simulink model "TestStructure"  (R2023b)
settings: Solver=FixedStepDiscrete  StartTime=0.0  StopTime=inf  FixedStep=SampleTime  RelTol=1e-3
InitFcn:
  | SampleTime = 0.001;
  | ButtonValue=0;
  | load("BusConfig.mat");
undefined symbols (not defined in the file): DiscIntNeverNeededParam
libraries: slrealtimeethercatlib x219, dspfdesign x28, dspstat3 x23, simulink x21, slpidlib x10, dspswit3 x8, commfilt2 x2, dspsigops x1
(part 6 of 8)

== system TestStructure/Bus/Subsystem6/Subsystem/Subsystem11 ==
  EtherCAT PDO Receive1 : slrealtimeethercatlib/EtherCAT PDO Receive  Priority=2  sig_name=Box 1 (PIC32 EtherCAT Slave01).INPUTS process data mapping.FORCE1  sig_offset=696  sig_type=single  type_size=32  sig_dim=1  device_id=0  sample_time=0.001000
  EtherCAT PDO Receive2 : slrealtimeethercatlib/EtherCAT PDO Receive  Priority=2  sig_name=Box 1 (PIC32 EtherCAT Slave01).INPUTS process data mapping.FORCE2  sig_offset=728  sig_type=single  type_size=32  sig_dim=1  device_id=0  sample_time=0.001000
  EtherCAT PDO Receive3 : slrealtimeethercatlib/EtherCAT PDO Receive  Priority=2  sig_name=Box 1 (PIC32 EtherCAT Slave01).INPUTS process data mapping.IMU1_X  sig_offset=952  sig_type=single  type_size=32  sig_dim=1  device_id=0  sample_time=0.001000
  EtherCAT PDO Receive4 : slrealtimeethercatlib/EtherCAT PDO Receive  Priority=2  sig_name=Box 1 (PIC32 EtherCAT Slave01).INPUTS process data mapping.IMU1_Y  sig_offset=984  sig_type=single  type_size=32  sig_dim=1  device_id=0  sample_time=0.001000
  EtherCAT PDO Receive5 : slrealtimeethercatlib/EtherCAT PDO Receive  Priority=2  sig_name=Box 1 (PIC32 EtherCAT Slave01).INPUTS process data mapping.IMU1_Z  sig_offset=1016  sig_type=single  type_size=32  sig_dim=1  device_id=0  sample_time=0.001000
  EtherCAT PDO Receive6 : slrealtimeethercatlib/EtherCAT PDO Receive  Priority=2  sig_name=Box 1 (PIC32 EtherCAT Slave01).INPUTS process data mapping.IMU2_X  sig_offset=1048  sig_type=single  type_size=32  sig_dim=1  device_id=0  sample_time=0.001000
  EtherCAT PDO Receive7 : slrealtimeethercatlib/EtherCAT PDO Receive  Priority=2  sig_name=Box 1 (PIC32 EtherCAT Slave01).INPUTS process data mapping.FORCE3  sig_offset=760  sig_type=single  type_size=32  sig_dim=1  device_id=0  sample_time=0.001000
  Out1 : Outport
  Out2 : Outport  Port=2
  Out3 : Outport  Port=3
  Out4 : Outport  Port=4
  Out5 : Outport  Port=5
  Out6 : Outport  Port=6
  Out7 : Outport  Port=7
  wires:
  EtherCAT PDO Receive1/1 -> Out1/1
  EtherCAT PDO Receive2/1 -> Out2/1
  EtherCAT PDO Receive3/1 -> Out3/1
  EtherCAT PDO Receive4/1 -> Out4/1
  EtherCAT PDO Receive5/1 -> Out5/1
  EtherCAT PDO Receive6/1 -> Out6/1
  EtherCAT PDO Receive7/1 -> Out7/1

== system TestStructure/Bus/Subsystem6/Subsystem/Subsystem2 ==
  In1 : Inport
  EtherCAT PDO Receive1 : slrealtimeethercatlib/EtherCAT PDO Receive  Priority=2  sig_name=Drive 6 (Elmo Drive ).Inputs.Position actual value  sig_offset=13232  sig_type=int32  type_size=32  sig_dim=1  device_id=0  sample_time=0.001000
  EtherCAT PDO Receive2 : slrealtimeethercatlib/EtherCAT PDO Receive  Priority=2  sig_name=Drive 6 (Elmo Drive ).Inputs_1.Velocity actual value  sig_offset=13312  sig_type=int32  type_size=32  sig_dim=1  device_id=0  sample_time=0.001000
  EtherCAT PDO Receive3 : slrealtimeethercatlib/EtherCAT PDO Receive  Priority=2  sig_name=Drive 6 (Elmo Drive ).Inputs.Torque actual value  sig_offset=13264  sig_type=int16  type_size=16  sig_dim=1  device_id=0  sample_time=0.001000
  EtherCAT PDO Receive4 : slrealtimeethercatlib/EtherCAT PDO Receive  Priority=2  sig_name=Drive 6 (Elmo Drive ).Inputs_2.DC link circuit voltage  sig_offset=13344  sig_type=uint32  type_size=32  sig_dim=1  device_id=0  sample_time=0.001000
  EtherCAT PDO Receive5 : slrealtimeethercatlib/EtherCAT PDO Receive  Priority=2  sig_name=Drive 6 (Elmo Drive ).Inputs.Mode of operation display  sig_offset=13296  sig_type=int8  type_size=8  sig_dim=1  device_id=0  sample_time=0.001000
  EtherCAT PDO Transmit : slrealtimeethercatlib/EtherCAT PDO Transmit  Priority=5  Commented=on  sig_name=Drive 4 (Elmo Drive ).Outputs.Target Torque  sig_offset=37072  sig_type=int16  type_size=16  sig_dim=1  device_id=0  sample_time=0.001000
  Out1 : Outport
  Out2 : Outport  Port=2
  Out3 : Outport  Port=3
  Out4 : Outport  Port=4
  Out5 : Outport  Port=5
  wires:
  In1/1 -> EtherCAT PDO Transmit/1
  EtherCAT PDO Receive5/1 -> Out5/1
  EtherCAT PDO Receive4/1 -> Out4/1
  EtherCAT PDO Receive3/1 -> Out3/1
  EtherCAT PDO Receive2/1 -> Out2/1
  EtherCAT PDO Receive1/1 -> Out1/1

== system TestStructure/Bus/Subsystem6/Subsystem/Subsystem3 ==
  In1 : Inport
  EtherCAT PDO Receive1 : slrealtimeethercatlib/EtherCAT PDO Receive  Priority=2  sig_name=Drive 2 (Elmo Drive ).Inputs.Position actual value  sig_offset=12496  sig_type=int32  type_size=32  sig_dim=1  device_id=0  sample_time=0.001000
  EtherCAT PDO Receive2 : slrealtimeethercatlib/EtherCAT PDO Receive  Priority=2  sig_name=Drive 2 (Elmo Drive ).Inputs_1.Velocity actual value  sig_offset=12576  sig_type=int32  type_size=32  sig_dim=1  device_id=0  sample_time=0.001000
  EtherCAT PDO Receive3 : slrealtimeethercatlib/EtherCAT PDO Receive  Priority=2  sig_name=Drive 2 (Elmo Drive ).Inputs.Torque actual value  sig_offset=12528  sig_type=int16  type_size=16  sig_dim=1  device_id=0  sample_time=0.001000
  EtherCAT PDO Receive4 : slrealtimeethercatlib/EtherCAT PDO Receive  Priority=2  sig_name=Drive 2 (Elmo Drive ).Inputs_2.DC link circuit voltage  sig_offset=12608  sig_type=uint32  type_size=32  sig_dim=1  device_id=0  sample_time=0.001000
  EtherCAT PDO Receive5 : slrealtimeethercatlib/EtherCAT PDO Receive  Priority=2  sig_name=Drive 2 (Elmo Drive ).Inputs.Mode of operation display  sig_offset=12560  sig_type=int8  type_size=8  sig_dim=1  device_id=0  sample_time=0.001000
  EtherCAT PDO Transmit : slrealtimeethercatlib/EtherCAT PDO Transmit  Priority=5  sig_name=Drive 2 (Elmo Drive ).Outputs.Target Torque  sig_offset=12496  sig_type=int16  type_size=16  sig_dim=1  device_id=0  sample_time=0.001000
  Out1 : Outport
  Out2 : Outport  Port=2
  Out3 : Outport  Port=3
  Out4 : Outport  Port=4
  Out5 : Outport  Port=5
  wires:
  In1/1 -> EtherCAT PDO Transmit/1
  EtherCAT PDO Receive5/1 -> Out5/1
  EtherCAT PDO Receive4/1 -> Out4/1
  EtherCAT PDO Receive3/1 -> Out3/1
  EtherCAT PDO Receive2/1 -> Out2/1
  EtherCAT PDO Receive1/1 -> Out1/1

== system TestStructure/Bus/Subsystem6/Subsystem/Subsystem4 ==
  In1 : Inport
  EtherCAT PDO Receive1 : slrealtimeethercatlib/EtherCAT PDO Receive  Priority=2  sig_name=Drive 2 (Elmo Drive ).Inputs.Position actual value  sig_offset=12496  sig_type=int32  type_size=32  sig_dim=1  device_id=0  sample_time=0.001000
  EtherCAT PDO Receive2 : slrealtimeethercatlib/EtherCAT PDO Receive  Priority=2  sig_name=Drive 2 (Elmo Drive ).Inputs_1.Velocity actual value  sig_offset=12576  sig_type=int32  type_size=32  sig_dim=1  device_id=0  sample_time=0.001000
  EtherCAT PDO Receive3 : slrealtimeethercatlib/EtherCAT PDO Receive  Priority=2  sig_name=Drive 2 (Elmo Drive ).Inputs.Torque actual value  sig_offset=12528  sig_type=int16  type_size=16  sig_dim=1  device_id=0  sample_time=0.001000
  EtherCAT PDO Receive4 : slrealtimeethercatlib/EtherCAT PDO Receive  Priority=2  sig_name=Drive 2 (Elmo Drive ).Inputs_2.DC link circuit voltage  sig_offset=12608  sig_type=uint32  type_size=32  sig_dim=1  device_id=0  sample_time=0.001000
  EtherCAT PDO Receive5 : slrealtimeethercatlib/EtherCAT PDO Receive  Priority=2  sig_name=Drive 2 (Elmo Drive ).Inputs.Mode of operation display  sig_offset=12560  sig_type=int8  type_size=8  sig_dim=1  device_id=0  sample_time=0.001000
  EtherCAT PDO Transmit : slrealtimeethercatlib/EtherCAT PDO Transmit  Priority=5  sig_name=Drive 2 (Elmo Drive ).Outputs.Target Torque  sig_offset=12496  sig_type=int16  type_size=16  sig_dim=1  device_id=0  sample_time=0.001000
  Out1 : Outport
  Out2 : Outport  Port=2
  Out3 : Outport  Port=3
  Out4 : Outport  Port=4
  Out5 : Outport  Port=5
  wires:
  In1/1 -> EtherCAT PDO Transmit/1
  EtherCAT PDO Receive5/1 -> Out5/1
  EtherCAT PDO Receive4/1 -> Out4/1
  EtherCAT PDO Receive3/1 -> Out3/1
  EtherCAT PDO Receive2/1 -> Out2/1
  EtherCAT PDO Receive1/1 -> Out1/1

== system TestStructure/Bus/Subsystem6/Subsystem/Subsystem5 ==
  EtherCAT PDO Receive1 : slrealtimeethercatlib/EtherCAT PDO Receive  Priority=2  sig_name=Box 2 (PIC32 EtherCAT Slave01).INPUTS process data mapping.FORCE1  sig_offset=696  sig_type=single  type_size=32  sig_dim=1  device_id=0  sample_time=0.001000
  EtherCAT PDO Receive{2..6} (5 alike) : slrealtimeethercatlib/EtherCAT PDO Receive  Priority=2  Commented=on  sig_name=Uninitialized Block  sig_offset=1  sig_type=boolean  type_size=1  sig_dim=1  device_id=0  sample_time=1
  EtherCAT PDO Receive7 : slrealtimeethercatlib/EtherCAT PDO Receive  Priority=2  sig_name=Box 2 (PIC32 EtherCAT Slave01).INPUTS process data mapping.FORCE3  sig_offset=760  sig_type=single  type_size=32  sig_dim=1  device_id=0  sample_time=0.001000
  Out1 : Outport
  Out2 : Outport  Port=2
  Out3 : Outport  Port=3
  Out4 : Outport  Port=4
  Out5 : Outport  Port=5
  Out6 : Outport  Port=6
  Out7 : Outport  Port=7
  wires:
  EtherCAT PDO Receive1/1 -> Out1/1
  EtherCAT PDO Receive2/1 -> Out2/1
  EtherCAT PDO Receive3/1 -> Out3/1
  EtherCAT PDO Receive4/1 -> Out4/1
  EtherCAT PDO Receive5/1 -> Out5/1
  EtherCAT PDO Receive6/1 -> Out6/1
  EtherCAT PDO Receive7/1 -> Out7/1

== system TestStructure/Bus/Subsystem6/Subsystem/Subsystem6 ==
  EtherCAT PDO Receive1 : slrealtimeethercatlib/EtherCAT PDO Receive  Priority=2  sig_name=Box 5 (PIC32 EtherCAT Slave01).INPUTS process data mapping.FORCE1  sig_offset=12496  sig_type=single  type_size=32  sig_dim=1  device_id=0  sample_time=0.001000
  EtherCAT PDO Receive2 : slrealtimeethercatlib/EtherCAT PDO Receive  Priority=2  Commented=on  sig_name=Box 6 (PIC32 EtherCAT Slave01).INPUTS process data mapping.FORCE2  sig_offset=37104  sig_type=single  type_size=32  sig_dim=1  device_id=0  sample_time=0.001000
  EtherCAT PDO Receive3 : slrealtimeethercatlib/EtherCAT PDO Receive  Priority=2  Commented=on  sig_name=Box 6 (PIC32 EtherCAT Slave01).INPUTS process data mapping.IMU1_X  sig_offset=37328  sig_type=single  type_size=32  sig_dim=1  device_id=0  sample_time=0.001000
  EtherCAT PDO Receive4 : slrealtimeethercatlib/EtherCAT PDO Receive  Priority=2  Commented=on  sig_name=Box 6 (PIC32 EtherCAT Slave01).INPUTS process data mapping.IMU1_Y  sig_offset=37360  sig_type=single  type_size=32  sig_dim=1  device_id=0  sample_time=0.001000
  EtherCAT PDO Receive5 : slrealtimeethercatlib/EtherCAT PDO Receive  Priority=2  Commented=on  sig_name=Box 6 (PIC32 EtherCAT Slave01).INPUTS process data mapping.IMU1_Z  sig_offset=37392  sig_type=single  type_size=32  sig_dim=1  device_id=0  sample_time=0.001000
  EtherCAT PDO Receive6 : slrealtimeethercatlib/EtherCAT PDO Receive  Priority=2  Commented=on  sig_name=Box 6 (PIC32 EtherCAT Slave01).INPUTS process data mapping.IMU2_X  sig_offset=37424  sig_type=single  type_size=32  sig_dim=1  device_id=0  sample_time=0.001000
  EtherCAT PDO Receive7 : slrealtimeethercatlib/EtherCAT PDO Receive  Priority=2  sig_name=Box 5 (PIC32 EtherCAT Slave01).INPUTS process data mapping.FORCE3  sig_offset=12560  sig_type=single  type_size=32  sig_dim=1  device_id=0  sample_time=0.001000
  Out1 : Outport
  Out2 : Outport  Port=2
  Out3 : Outport  Port=3
  Out4 : Outport  Port=4
  Out5 : Outport  Port=5
  Out6 : Outport  Port=6
  Out7 : Outport  Port=7
  wires:
  EtherCAT PDO Receive1/1 -> Out1/1
  EtherCAT PDO Receive2/1 -> Out2/1
  EtherCAT PDO Receive3/1 -> Out3/1
  EtherCAT PDO Receive4/1 -> Out4/1
  EtherCAT PDO Receive5/1 -> Out5/1
  EtherCAT PDO Receive6/1 -> Out6/1
  EtherCAT PDO Receive7/1 -> Out7/1

== system TestStructure/Bus/Subsystem6/Subsystem/Subsystem7 ==
  EtherCAT PDO Receive1 : slrealtimeethercatlib/EtherCAT PDO Receive  Priority=2  sig_name=Box 1 (PIC32 EtherCAT Slave01).INPUTS process data mapping.FORCE1  sig_offset=696  sig_type=single  type_size=32  sig_dim=1  device_id=0  sample_time=0.001000
  EtherCAT PDO Receive2 : slrealtimeethercatlib/EtherCAT PDO Receive  Priority=2  sig_name=Box 1 (PIC32 EtherCAT Slave01).INPUTS process data mapping.FORCE2  sig_offset=728  sig_type=single  type_size=32  sig_dim=1  device_id=0  sample_time=0.001000
  EtherCAT PDO Receive3 : slrealtimeethercatlib/EtherCAT PDO Receive  Priority=2  sig_name=Box 1 (PIC32 EtherCAT Slave01).INPUTS process data mapping.IMU1_X  sig_offset=952  sig_type=single  type_size=32  sig_dim=1  device_id=0  sample_time=0.001000
  EtherCAT PDO Receive4 : slrealtimeethercatlib/EtherCAT PDO Receive  Priority=2  sig_name=Box 1 (PIC32 EtherCAT Slave01).INPUTS process data mapping.IMU1_Y  sig_offset=984  sig_type=single  type_size=32  sig_dim=1  device_id=0  sample_time=0.001000
  EtherCAT PDO Receive5 : slrealtimeethercatlib/EtherCAT PDO Receive  Priority=2  sig_name=Box 1 (PIC32 EtherCAT Slave01).INPUTS process data mapping.IMU1_Z  sig_offset=1016  sig_type=single  type_size=32  sig_dim=1  device_id=0  sample_time=0.001000
  EtherCAT PDO Receive6 : slrealtimeethercatlib/EtherCAT PDO Receive  Priority=2  sig_name=Box 1 (PIC32 EtherCAT Slave01).INPUTS process data mapping.IMU2_X  sig_offset=1048  sig_type=single  type_size=32  sig_dim=1  device_id=0  sample_time=0.001000
  EtherCAT PDO Receive7 : slrealtimeethercatlib/EtherCAT PDO Receive  Priority=2  sig_name=Box 1 (PIC32 EtherCAT Slave01).INPUTS process data mapping.FORCE3  sig_offset=760  sig_type=single  type_size=32  sig_dim=1  device_id=0  sample_time=0.001000
  Out1 : Outport
  Out2 : Outport  Port=2
  Out3 : Outport  Port=3
  Out4 : Outport  Port=4
  Out5 : Outport  Port=5
  Out6 : Outport  Port=6
  Out7 : Outport  Port=7
  wires:
  EtherCAT PDO Receive1/1 -> Out1/1
  EtherCAT PDO Receive2/1 -> Out2/1
  EtherCAT PDO Receive3/1 -> Out3/1
  EtherCAT PDO Receive4/1 -> Out4/1
  EtherCAT PDO Receive5/1 -> Out5/1
  EtherCAT PDO Receive6/1 -> Out6/1
  EtherCAT PDO Receive7/1 -> Out7/1

== system TestStructure/Bus/Subsystem6/Subsystem/Subsystem8 ==
  EtherCAT PDO Receive1 : slrealtimeethercatlib/EtherCAT PDO Receive  Priority=2  sig_name=Box 1 (PIC32 EtherCAT Slave01).INPUTS process data mapping.FORCE1  sig_offset=696  sig_type=single  type_size=32  sig_dim=1  device_id=0  sample_time=0.001000
  EtherCAT PDO Receive2 : slrealtimeethercatlib/EtherCAT PDO Receive  Priority=2  sig_name=Box 1 (PIC32 EtherCAT Slave01).INPUTS process data mapping.FORCE2  sig_offset=728  sig_type=single  type_size=32  sig_dim=1  device_id=0  sample_time=0.001000
  EtherCAT PDO Receive3 : slrealtimeethercatlib/EtherCAT PDO Receive  Priority=2  sig_name=Box 1 (PIC32 EtherCAT Slave01).INPUTS process data mapping.IMU1_X  sig_offset=952  sig_type=single  type_size=32  sig_dim=1  device_id=0  sample_time=0.001000
  EtherCAT PDO Receive4 : slrealtimeethercatlib/EtherCAT PDO Receive  Priority=2  sig_name=Box 1 (PIC32 EtherCAT Slave01).INPUTS process data mapping.IMU1_Y  sig_offset=984  sig_type=single  type_size=32  sig_dim=1  device_id=0  sample_time=0.001000
  EtherCAT PDO Receive5 : slrealtimeethercatlib/EtherCAT PDO Receive  Priority=2  sig_name=Box 1 (PIC32 EtherCAT Slave01).INPUTS process data mapping.IMU1_Z  sig_offset=1016  sig_type=single  type_size=32  sig_dim=1  device_id=0  sample_time=0.001000
  EtherCAT PDO Receive6 : slrealtimeethercatlib/EtherCAT PDO Receive  Priority=2  sig_name=Box 1 (PIC32 EtherCAT Slave01).INPUTS process data mapping.IMU2_X  sig_offset=1048  sig_type=single  type_size=32  sig_dim=1  device_id=0  sample_time=0.001000
  EtherCAT PDO Receive7 : slrealtimeethercatlib/EtherCAT PDO Receive  Priority=2  sig_name=Box 1 (PIC32 EtherCAT Slave01).INPUTS process data mapping.FORCE3  sig_offset=760  sig_type=single  type_size=32  sig_dim=1  device_id=0  sample_time=0.001000
  Out1 : Outport
  Out2 : Outport  Port=2
  Out3 : Outport  Port=3
  Out4 : Outport  Port=4
  Out5 : Outport  Port=5
  Out6 : Outport  Port=6
  Out7 : Outport  Port=7
  wires:
  EtherCAT PDO Receive1/1 -> Out1/1
  EtherCAT PDO Receive2/1 -> Out2/1
  EtherCAT PDO Receive3/1 -> Out3/1
  EtherCAT PDO Receive4/1 -> Out4/1
  EtherCAT PDO Receive5/1 -> Out5/1
  EtherCAT PDO Receive6/1 -> Out6/1
  EtherCAT PDO Receive7/1 -> Out7/1

== system TestStructure/Bus/Subsystem6/Subsystem/Subsystem9 ==
  EtherCAT PDO Receive1 : slrealtimeethercatlib/EtherCAT PDO Receive  Priority=2  sig_name=Box 1 (PIC32 EtherCAT Slave01).INPUTS process data mapping.FORCE1  sig_offset=696  sig_type=single  type_size=32  sig_dim=1  device_id=0  sample_time=0.001000
  EtherCAT PDO Receive2 : slrealtimeethercatlib/EtherCAT PDO Receive  Priority=2  sig_name=Box 1 (PIC32 EtherCAT Slave01).INPUTS process data mapping.FORCE2  sig_offset=728  sig_type=single  type_size=32  sig_dim=1  device_id=0  sample_time=0.001000
  EtherCAT PDO Receive3 : slrealtimeethercatlib/EtherCAT PDO Receive  Priority=2  sig_name=Box 1 (PIC32 EtherCAT Slave01).INPUTS process data mapping.IMU1_X  sig_offset=952  sig_type=single  type_size=32  sig_dim=1  device_id=0  sample_time=0.001000
  EtherCAT PDO Receive4 : slrealtimeethercatlib/EtherCAT PDO Receive  Priority=2  sig_name=Box 1 (PIC32 EtherCAT Slave01).INPUTS process data mapping.IMU1_Y  sig_offset=984  sig_type=single  type_size=32  sig_dim=1  device_id=0  sample_time=0.001000
  EtherCAT PDO Receive5 : slrealtimeethercatlib/EtherCAT PDO Receive  Priority=2  sig_name=Box 1 (PIC32 EtherCAT Slave01).INPUTS process data mapping.IMU1_Z  sig_offset=1016  sig_type=single  type_size=32  sig_dim=1  device_id=0  sample_time=0.001000
  EtherCAT PDO Receive6 : slrealtimeethercatlib/EtherCAT PDO Receive  Priority=2  sig_name=Box 1 (PIC32 EtherCAT Slave01).INPUTS process data mapping.IMU2_X  sig_offset=1048  sig_type=single  type_size=32  sig_dim=1  device_id=0  sample_time=0.001000
  EtherCAT PDO Receive7 : slrealtimeethercatlib/EtherCAT PDO Receive  Priority=2  sig_name=Box 1 (PIC32 EtherCAT Slave01).INPUTS process data mapping.FORCE3  sig_offset=760  sig_type=single  type_size=32  sig_dim=1  device_id=0  sample_time=0.001000
  Out1 : Outport
  Out2 : Outport  Port=2
  Out3 : Outport  Port=3
  Out4 : Outport  Port=4
  Out5 : Outport  Port=5
  Out6 : Outport  Port=6
  Out7 : Outport  Port=7
  wires:
  EtherCAT PDO Receive1/1 -> Out1/1
  EtherCAT PDO Receive2/1 -> Out2/1
  EtherCAT PDO Receive3/1 -> Out3/1
  EtherCAT PDO Receive4/1 -> Out4/1
  EtherCAT PDO Receive5/1 -> Out5/1
  EtherCAT PDO Receive6/1 -> Out6/1
  EtherCAT PDO Receive7/1 -> Out7/1

== system TestStructure/Bus/Subsystem6/Subsystem2/Subsystem7 ==
  EtherCAT PDO Receive1 : slrealtimeethercatlib/EtherCAT PDO Receive  Priority=2  sig_name=Box 8 (PIC32 EtherCAT Slave01).INPUTS process data mapping.FORCE1  sig_offset=24784  sig_type=single  type_size=32  sig_dim=1  device_id=0  sample_time=0.001000
  EtherCAT PDO Receive2 : slrealtimeethercatlib/EtherCAT PDO Receive  Priority=2  sig_name=Box 8 (PIC32 EtherCAT Slave01).INPUTS process data mapping.FORCE2  sig_offset=24816  sig_type=single  type_size=32  sig_dim=1  device_id=0  sample_time=0.001000
  EtherCAT PDO Receive3 : slrealtimeethercatlib/EtherCAT PDO Receive  Priority=2  sig_name=Box 8 (PIC32 EtherCAT Slave01).INPUTS process data mapping.FORCE3  sig_offset=24848  sig_type=single  type_size=32  sig_dim=1  device_id=0  sample_time=0.001000
  EtherCAT PDO Receive4 : slrealtimeethercatlib/EtherCAT PDO Receive  Priority=2  sig_name=Box 8 (PIC32 EtherCAT Slave01).INPUTS process data mapping.FORCE4  sig_offset=24880  sig_type=single  type_size=32  sig_dim=1  device_id=0  sample_time=0.001000
  EtherCAT PDO Receive7 : slrealtimeethercatlib/EtherCAT PDO Receive  Priority=2  Commented=on  sig_name=Box 2 (PIC32 EtherCAT Slave01).INPUTS process data mapping.FORCE5  sig_offset=824  sig_type=single  type_size=32  sig_dim=1  device_id=0  sample_time=0.001000
  Out1 : Outport
  Out2 : Outport  Port=2
  Out3 : Outport  Port=3
  Out4 : Outport  Port=4
  Out7 : Outport  Port=5
  wires:
  EtherCAT PDO Receive1/1 -> Out1/1
  EtherCAT PDO Receive2/1 -> Out2/1
  EtherCAT PDO Receive3/1 -> Out3/1
  EtherCAT PDO Receive4/1 -> Out4/1
  EtherCAT PDO Receive7/1 -> Out7/1

== system TestStructure/Bus/Subsystem6/Subsystem2/Subsystem8 ==
  EtherCAT PDO Receive1 : slrealtimeethercatlib/EtherCAT PDO Receive  Priority=2  sig_name=Box 9 (PIC32 EtherCAT Slave01).INPUTS process data mapping.FORCE1  sig_offset=37072  sig_type=single  type_size=32  sig_dim=1  device_id=0  sample_time=0.001000
  EtherCAT PDO Receive2 : slrealtimeethercatlib/EtherCAT PDO Receive  Priority=2  sig_name=Box 9 (PIC32 EtherCAT Slave01).INPUTS process data mapping.FORCE2  sig_offset=37104  sig_type=single  type_size=32  sig_dim=1  device_id=0  sample_time=0.001000
  EtherCAT PDO Receive3 : slrealtimeethercatlib/EtherCAT PDO Receive  Priority=2  sig_name=Box 9 (PIC32 EtherCAT Slave01).INPUTS process data mapping.FORCE3  sig_offset=37136  sig_type=single  type_size=32  sig_dim=1  device_id=0  sample_time=0.001000
  EtherCAT PDO Receive4 : slrealtimeethercatlib/EtherCAT PDO Receive  Priority=2  sig_name=Box 9 (PIC32 EtherCAT Slave01).INPUTS process data mapping.FORCE4  sig_offset=37168  sig_type=single  type_size=32  sig_dim=1  device_id=0  sample_time=0.001000
  EtherCAT PDO Receive7 : slrealtimeethercatlib/EtherCAT PDO Receive  Priority=2  Commented=on  sig_name=Box 3 (PIC32 EtherCAT Slave01).INPUTS process data mapping.FORCE5  sig_offset=24912  sig_type=single  type_size=32  sig_dim=1  device_id=0  sample_time=0.001000
  Out1 : Outport
  Out2 : Outport  Port=2
  Out3 : Outport  Port=3
  Out4 : Outport  Port=4
  Out7 : Outport  Port=5
  wires:
  EtherCAT PDO Receive1/1 -> Out1/1
  EtherCAT PDO Receive2/1 -> Out2/1
  EtherCAT PDO Receive3/1 -> Out3/1
  EtherCAT PDO Receive4/1 -> Out4/1
  EtherCAT PDO Receive7/1 -> Out7/1

== system TestStructure/InterForceControlTask/AO/PhaseCorrection/If Action Subsystem ==
  Action Port : ActionPort  ActionPortLabel=if(u1 == 1)
  Constant : Constant
  Out1 : Outport
  wires:
  Constant/1 -> Out1/1

== system TestStructure/InterForceControlTask/AO/PhaseCorrection/If Action Subsystem1 ==
  Action Port : ActionPort  ActionPortLabel=else
  Constant : Constant  Value=0
  Out1 : Outport
  wires:
  Constant/1 -> Out1/1

== system TestStructure/InterForceControlTask/AO/Select/If Action Subsystem ==
  Phi : Inport
  Phase0 : Inport  Port=2
  Action Port : ActionPort  InitializeStates=reset  ActionPortLabel=else
  Constant1 : Constant
  Counter1 : dspswit3/Counter  Direction=Up  CountEvent=Rising edge  CounterSize=8 bits  MaxCount=255  InitialCount=0  Output=Count  HitValue=32  ResetInput=off  SamplesPerFrame=1  Ts=1  CntDtype=double  HitDtype=Logical
  If : If
  If Action Subsystem : Subsystem  TreatAsAtomicUnit=on
  If Action Subsystem1 : Subsystem  TreatAsAtomicUnit=on
  Merge : Merge
  Merge1 : Merge
  Phi_Out : Outport
  Phase0Event : Outport  Port=2
  En : Outport  Port=3
  wires:
  Constant1/1 -> En/1
  Phase0/1 -> If Action Subsystem/2(Phase0), Counter1/1
  Phi/1 -> If Action Subsystem/1(Phi)
  Counter1/1 -> If/1
  Merge/1 -> Phi_Out/1
  If/1 -> If Action Subsystem/Action
  If Action Subsystem/1(Out1) -> Merge/1
  If/2 -> If Action Subsystem1/Action
  If Action Subsystem1/1(Out1) -> Merge/2
  Merge1/1 -> Phase0Event/1
  If Action Subsystem1/2(Out2) -> Merge1/2
  If Action Subsystem/2(Out2) -> Merge1/1

== system TestStructure/InterForceControlTask/AO/Select/If Action Subsystem1 ==
  Action Port : ActionPort  ActionPortLabel=if((u1 >= 10.5)|(u2 <= u3))
  Constant : Constant  Value=0
  Constant1 : Constant  Value=0
  Constant2 : Constant  Value=0
  Out1 : Outport
  Out2 : Outport  Port=2
  Out3 : Outport  Port=3
  wires:
  Constant2/1 -> Out3/1
  Constant1/1 -> Out2/1
  Constant/1 -> Out1/1

== system TestStructure/InterForceControlTask/AO/Subsystem1/Abs-based selector ==
  candidate : Inport
  Constant2 : Constant  Value=0
  Constant4 : Constant  Value=0
  Gain1 : Gain  Gain=-1
  MATLAB Function : MATLAB Function  TreatAsAtomicUnit=on
  Moving Maximum1 : dspstat3/Moving Maximum  SpecifyWindowLength=on  WindowLength=2000  SimulateUsing=Code generation
  Moving Maximum2 : dspstat3/Moving Maximum  SpecifyWindowLength=on  WindowLength=2000  SimulateUsing=Code generation
  Switch1 : Switch  Criteria=u2 > Threshold  SaturateOnIntegerOverflow=off  InputSameDT=off
  Switch2 : Switch  Criteria=u2 > Threshold  SaturateOnIntegerOverflow=off  InputSameDT=off
  mode : Outport
  wires:
  Moving Maximum2/1 -> MATLAB Function/3(neg_env)
  Gain1/1 -> Switch2/2, Switch2/1
  Constant2/1 -> Switch1/3
  Switch1/1 -> Moving Maximum1/1  "pos_amp"
  Switch2/1 -> Moving Maximum2/1  "neg_amp"
  candidate/1 -> Gain1/1, Switch1/2, Switch1/1, MATLAB Function/1(candidate)
  Constant4/1 -> Switch2/3
  Moving Maximum1/1 -> MATLAB Function/2(pos_env)
  MATLAB Function/1(mode) -> mode/1

== system TestStructure/InterForceControlTask/AO/Subsystem1/Detector1 ==
  p8 : Inport  PortDimensions=8
  Whichfoot : Inport  Port=2
  Constant : Constant  Value=true
  ContactRelay : Relay  OnSwitchValue=2.0  OffSwitchValue=1.25
  EventAndStartupGate : Logic  AllPortsSameDT=off  OutDataTypeStr=boolean
  EventToDouble : DataTypeConversion  OutDataTypeStr=double  SaturateOnIntegerOverflow=off  RndMeth=Floor
  LeftLowPass : DiscreteTransferFcn  Numerator=0.05  Denominator=[1 -0.95]  SampleTime=0.001
  PrevContact : UnitDelay  SampleTime=0.001  HasFrameUpgradeWarning=on
  RisingEdge : RelationalOperator  Operator=>  OutDataTypeStr=boolean  RndMeth=Simplest  InputSameDT=off
  Switch : Switch  Criteria=u2 > Threshold  SaturateOnIntegerOverflow=off  InputSameDT=off
  VoltageToFootLoad : MATLAB Function  TreatAsAtomicUnit=on
  Phase0Event : Outport
  LeftLoad : Outport  Port=2
  RightLoad : Outport  Port=3
  wires:
  p8/1 -> VoltageToFootLoad/1(p8)
  VoltageToFootLoad/1(leftLoad) -> Switch/1, LeftLoad/1
  LeftLowPass/1 -> ContactRelay/1
  ContactRelay/1 -> RisingEdge/1, PrevContact/1
  PrevContact/1 -> RisingEdge/2
  RisingEdge/1 -> EventAndStartupGate/1
  Constant/1 -> EventAndStartupGate/2
  EventAndStartupGate/1 -> EventToDouble/1
  EventToDouble/1 -> Phase0Event/1
  VoltageToFootLoad/2(rightLoad) -> Switch/3, RightLoad/1
  Whichfoot/1 -> Switch/2
  Switch/1 -> LeftLowPass/1

== system TestStructure/InterForceControlTask/AO/Subsystem1/Function-Call Subsystem ==
  Action Port : ActionPort  ActionPortLabel=if((u1 > u2))
  Constant : Constant
  Out1 : Outport
  wires:
  Constant/1 -> Out1/1

== system TestStructure/InterForceControlTask/AO/Subsystem1/Function-Call Subsystem1 ==
  Action Port : ActionPort  ActionPortLabel=else
  Constant : Constant  Value=0
  Out1 : Outport
  wires:
  Constant/1 -> Out1/1

== system TestStructure/InterForceControlTask/AO/Subsystem1/Function-Call Subsystem2 ==
  Action Port : ActionPort  ActionPortLabel=elseif((u1< -u2))
  Constant : Constant  Value=-1
  Out1 : Outport
  wires:
  Constant/1 -> Out1/1

== system TestStructure/InterForceControlTask/AO/Subsystem1/If Action Subsystem ==
  Action Port : ActionPort  ActionPortLabel=if(u1 == 1)
  Constant : Constant
  Out1 : Outport
  wires:
  Constant/1 -> Out1/1

== system TestStructure/InterForceControlTask/AO/Subsystem1/If Action Subsystem1 ==
  Action Port : ActionPort  ActionPortLabel=else
  Constant : Constant  Value=0
  Out1 : Outport
  wires:
  Constant/1 -> Out1/1

== system TestStructure/InterForceControlTask/AO/Subsystem1/If Action Subsystem2 ==
  WindowMin : Inport
  threadhold : Inport  Port=2
  Action Port : ActionPort  ActionPortLabel=if((u1 > -0.02)&(u1<0.02))
  Constant : Constant
  Function-Call Subsystem : Subsystem  TreatAsAtomicUnit=on
  Function-Call Subsystem1 : Subsystem  TreatAsAtomicUnit=on
  Function-Call Subsystem2 : Subsystem  TreatAsAtomicUnit=on
  If : If  IfExpression=(u1 > 0.4)  ElseIfExpressions=(u1< -0.4)
  MATLAB Function1 : MATLAB Function  TreatAsAtomicUnit=on
  Merge : Merge  Inputs=3
  Out1 : Outport
  Out2 : Outport  Port=2
  y : Outport  Port=3
  wires:
  If/1 -> Function-Call Subsystem/Action
  Merge/1 -> Out1/1
  Function-Call Subsystem/1(Out1) -> Merge/1  "1"
  Function-Call Subsystem1/1(Out1) -> Merge/3  "0"
  WindowMin/1 -> MATLAB Function1/1(u)
  If/3 -> Function-Call Subsystem1/Action
  If/2 -> Function-Call Subsystem2/Action
  Function-Call Subsystem2/1(Out1) -> Merge/2  "-1"
  MATLAB Function1/1(y) -> y/1, If/1
  Constant/1 -> Out2/1
  threadhold/1 -> MATLAB Function1/2(threadhold)

== system TestStructure/InterForceControlTask/AO/Subsystem1/If Action Subsystem3 ==
  Action Port : ActionPort  ActionPortLabel=else
  Constant : Constant  Value=0
  Constant1 : Constant  Value=0
  Out1 : Outport
  Out2 : Outport  Port=2
  wires:
  Constant/1 -> Out1/1
  Constant1/1 -> Out2/1

== system TestStructure/InterForceControlTask/AO/Subsystem1/Triggered Subsystem ==
  In1 : Inport
  Trigger : TriggerPort  VariantControl=(inherit)
  t-t_start : Outport
  wires:
  In1/1 -> t-t_start/1

== system TestStructure/InterForceControlTask/AO1/PhaseCorrection/If Action Subsystem ==
  Action Port : ActionPort
  Constant : Constant
  Out1 : Outport
  wires:
  Constant/1 -> Out1/1

== system TestStructure/InterForceControlTask/AO1/PhaseCorrection/If Action Subsystem1 ==
  Action Port : ActionPort
  Constant : Constant  Value=0
  Out1 : Outport
  wires:
  Constant/1 -> Out1/1

== system TestStructure/InterForceControlTask/AO1/Select/If Action Subsystem ==
  Phi : Inport
  Phase0 : Inport  Port=2
  Action Port : ActionPort  InitializeStates=reset
  Constant1 : Constant
  Counter1 : dspswit3/Counter  Direction=Up  CountEvent=Rising edge  CounterSize=8 bits  MaxCount=255  InitialCount=0  Output=Count  HitValue=32  ResetInput=off  SamplesPerFrame=1  Ts=1  CntDtype=double  HitDtype=Logical
  If : If
  If Action Subsystem : Subsystem  TreatAsAtomicUnit=on
  If Action Subsystem1 : Subsystem  TreatAsAtomicUnit=on
  Merge : Merge
  Merge1 : Merge
  Phi_Out : Outport
  Phase0Event : Outport  Port=2
  En : Outport  Port=3
  wires:
  Constant1/1 -> En/1
  Phase0/1 -> If Action Subsystem/2(Phase0), Counter1/1
  Phi/1 -> If Action Subsystem/1(Phi)
  Counter1/1 -> If/1
  Merge/1 -> Phi_Out/1
  If/1 -> If Action Subsystem/Action
  If Action Subsystem/1(Out1) -> Merge/1
  If/2 -> If Action Subsystem1/Action
  If Action Subsystem1/1(Out1) -> Merge/2
  Merge1/1 -> Phase0Event/1
  If Action Subsystem1/2(Out2) -> Merge1/2
  If Action Subsystem/2(Out2) -> Merge1/1

== system TestStructure/InterForceControlTask/AO1/Select/If Action Subsystem1 ==
  Action Port : ActionPort
  Constant : Constant  Value=0
  Constant1 : Constant  Value=0
  Constant2 : Constant  Value=0
  Out1 : Outport
  Out2 : Outport  Port=2
  Out3 : Outport  Port=3
  wires:
  Constant2/1 -> Out3/1
  Constant1/1 -> Out2/1
  Constant/1 -> Out1/1

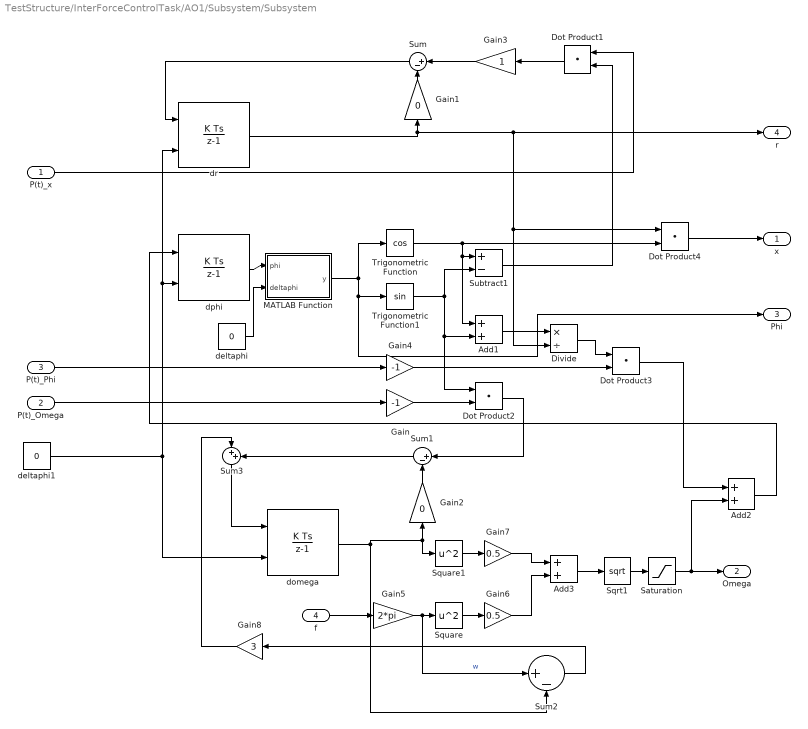
== system TestStructure/InterForceControlTask/AO1/Subsystem/Subsystem ==
  P(t)_x : Inport
  P(t)_Omega : Inport  Port=2
  P(t)_Phi : Inport  Port=3
  f : Inport  Port=4
  Add1 : Sum
  Add2 : Sum
  Add3 : Sum
  Divide : Product  Inputs=*/
  Dot Product{1..4} (4 alike) : DotProduct  OutDataTypeStr=Inherit: Inherit via internal rule
  Gain : Gain  Gain=-1
  Gain1 : Gain  Gain=0
  Gain2 : Gain  Gain=0
  Gain3 : Gain
  Gain4 : Gain  Gain=-1
  Gain5 : Gain  Gain=2*pi
  Gain6 : Gain  Gain=0.5
  Gain7 : Gain  Gain=0.5
  Gain8 : Gain  Gain=3
  MATLAB Function : MATLAB Function  TreatAsAtomicUnit=on
  Saturation : Saturate  UpperLimit=2*pi*1  LowerLimit=2*pi*0.15
  Sqrt1 : Sqrt
  Square : Math  Operator=square
  Square1 : Math  Operator=square
  Subtract1 : Sum  Inputs=+-
  Sum : Sum  Inputs=|+-
  Sum1 : Sum  Inputs=|+-
  Sum2 : Sum  Inputs=|+-
  Sum3 : Sum  Inputs=|++
  Trigonometric Function : Trigonometry  Operator=cos
  Trigonometric Function1 : Trigonometry
  deltaphi : Constant  Value=0
  deltaphi1 : Constant  Value=0
  domega : DiscreteIntegrator  ExternalReset=falling  InitialCondition=0.3*2*pi  SampleTime=-1  LimitOutput=on  UpperSaturationLimit=2*pi*0.9  LowerSaturationLimit=2*pi*0.15  ICPrevOutput=DiscIntNeverNeededParam  ICPrevScaledInput=DiscIntNeverNeededParam
  dphi : DiscreteIntegrator  ExternalReset=falling  InitialCondition=1  SampleTime=-1  ICPrevOutput=DiscIntNeverNeededParam  ICPrevScaledInput=DiscIntNeverNeededParam
  dr : DiscreteIntegrator  ExternalReset=falling  InitialCondition=1  SampleTime=-1  ICPrevOutput=DiscIntNeverNeededParam  ICPrevScaledInput=DiscIntNeverNeededParam
  x : Outport
  Omega : Outport  Port=2
  Phi : Outport  Port=3
  r : Outport  Port=4
  wires:
  Gain8/1 -> Sum3/1
  Sum3/1 -> domega/1
  Sum2/1 -> Gain8/1
  Gain6/1 -> Add3/2
  Gain7/1 -> Add3/1
  domega/1 -> Sum2/2, Gain2/1, Square1/1
  Square1/1 -> Gain7/1
  f/1 -> Gain5/1
  Square/1 -> Gain6/1
  Gain5/1 -> Square/1, Sum2/1  "w"
  Saturation/1 -> Omega/1, Add2/2
  Sqrt1/1 -> Saturation/1
  Add3/1 -> Sqrt1/1
  Gain4/1 -> Dot Product3/2
  P(t)_Omega/1 -> Gain/1
  P(t)_x/1 -> Dot Product1/1
  P(t)_Phi/1 -> Gain4/1
  Trigonometric Function/1 -> Dot Product4/2, Subtract1/1, Add1/1
  deltaphi1/1 -> domega/2, dphi/2, dr/2
  Gain3/1 -> Sum/1
  Sum/1 -> dr/1
  Gain2/1 -> Sum1/2
  Sum1/1 -> Sum3/2
  Gain1/1 -> Sum/2
  dr/1 -> r/1, Dot Product4/1, Divide/2, Gain1/1
  deltaphi/1 -> MATLAB Function/2(deltaphi)
  dphi/1 -> MATLAB Function/1(phi)
  Divide/1 -> Dot Product3/1
  Subtract1/1 -> Dot Product1/2
  Dot Product3/1 -> Add2/1
  Dot Product1/1 -> Gain3/1
  Trigonometric Function1/1 -> Dot Product2/1, Add1/2, Subtract1/2
  Dot Product4/1 -> x/1
  Gain/1 -> Dot Product2/2
  Dot Product2/1 -> Sum1/1
  MATLAB Function/1(y) -> Trigonometric Function1/1, Phi/1, Trigonometric Function/1
  Add1/1 -> Divide/1
  Add2/1 -> dphi/1

== system TestStructure/InterForceControlTask/AO1/Subsystem/Subsystem1 ==
  P(t)_x : Inport
  P(t)_Phi : Inport  Port=2
  Omega : Inport  Port=3
  Add1 : Sum
  Add2 : Sum
  Divide : Product  Inputs=*/
  Dot Product1 : DotProduct  OutDataTypeStr=Inherit: Inherit via internal rule
  Dot Product3 : DotProduct  OutDataTypeStr=Inherit: Inherit via internal rule
  Dot Product4 : DotProduct  OutDataTypeStr=Inherit: Inherit via internal rule
  Gain : Gain  Gain=2
  Gain1 : Gain  Gain=0
  Gain3 : Gain
  Gain4 : Gain  Gain=-1
  MATLAB Function : MATLAB Function  TreatAsAtomicUnit=on
  Subtract1 : Sum  Inputs=+-
  Sum : Sum  Inputs=|+-
  Trigonometric Function : Trigonometry  Operator=cos
  Trigonometric Function1 : Trigonometry
  deltaphi : Constant  Value=0
  deltaphi1 : Constant  Value=0
  dphi : DiscreteIntegrator  ExternalReset=falling  InitialCondition=1  SampleTime=-1  ICPrevOutput=DiscIntNeverNeededParam  ICPrevScaledInput=DiscIntNeverNeededParam
  dr : DiscreteIntegrator  ExternalReset=falling  InitialCondition=1  SampleTime=-1  ICPrevOutput=DiscIntNeverNeededParam  ICPrevScaledInput=DiscIntNeverNeededParam
  x : Outport
  Phi : Outport  Port=2
  r : Outport  Port=3
  wires:
  Gain/1 -> Add2/2
  Gain4/1 -> Dot Product3/2
  P(t)_x/1 -> Dot Product1/1
  P(t)_Phi/1 -> Gain4/1
  Trigonometric Function/1 -> Dot Product4/2, Subtract1/1, Add1/1
  deltaphi1/1 -> dphi/2, dr/2
  Gain3/1 -> Sum/1
  Sum/1 -> dr/1
  Gain1/1 -> Sum/2
  dr/1 -> Gain1/1, r/1, Dot Product4/1, Divide/2
  deltaphi/1 -> MATLAB Function/2(deltaphi)
  dphi/1 -> MATLAB Function/1(phi)
  Divide/1 -> Dot Product3/1
  Subtract1/1 -> Dot Product1/2
  Dot Product3/1 -> Add2/1
  Dot Product1/1 -> Gain3/1
  Omega/1 -> Gain/1
  Trigonometric Function1/1 -> Add1/2, Subtract1/2
  Dot Product4/1 -> x/1
  MATLAB Function/1(y) -> Trigonometric Function1/1, Phi/1, Trigonometric Function/1
  Add1/1 -> Divide/1
  Add2/1 -> dphi/1

== system TestStructure/InterForceControlTask/AO1/Subsystem/Subsystem2 ==
  note: 交替打腿 7.5 0.7
  T(t) : Inport
  X(t) : Inport  Port=2
  Reset : Inport  Port=3
  0.1 : Gain  Gain=12
  0.2 : Gain  Gain=60
  0.3 : Gain  Gain=10
  0.4 : Gain  Gain=4
  Abs : Abs  SaturateOnIntegerOverflow=off
  Abs1 : Abs  SaturateOnIntegerOverflow=off
  Add3 : Sum  Inputs=+-+
  Add4 : Sum  Inputs=+-+
  Discrete Derivative : simulink/Discrete/Discrete Derivative  gainval=1.0  ICPrevScaledInput=0.0  OutMin=[]  OutMax=[]  OutDataType=fixdt(1, 16)  OutScaling=2^-10  DoSatur=off
  Discrete Derivative1 : simulink/Discrete/Discrete Derivative  gainval=1.0  ICPrevScaledInput=0.0  OutMin=[]  OutMax=[]  OutDataType=fixdt(1, 16)  OutScaling=2^-10  DoSatur=off
  Discrete-Time Integrator3 : DiscreteIntegrator  ExternalReset=falling  InitialCondition=0.1  SampleTime=-1  ICPrevOutput=DiscIntNeverNeededParam  ICPrevScaledInput=DiscIntNeverNeededParam
  Discrete-Time Integrator4 : DiscreteIntegrator  ExternalReset=falling  InitialCondition=0.01  SampleTime=-1  ICPrevOutput=DiscIntNeverNeededParam  ICPrevScaledInput=DiscIntNeverNeededParam
  Dot Product{1..3,5..7,10} (7 alike) : DotProduct  OutDataTypeStr=Inherit: Inherit via internal rule
  Gain : Gain  Gain=10
  Gain1 : Gain  Gain=3
  Saturation : Saturate  UpperLimit=40  LowerLimit=0
  Saturation3 : Saturate  UpperLimit=40  LowerLimit=0
  Subtract2 : Sum
  Sum1 : Sum  Inputs=-+|
  Sum2 : Sum  Inputs=-+|
  amp1 : Gain
  amp2 : Gain
  eta_0 : Constant  Value=2
  eta_1 : Constant
  eta_2 : Constant  Value=20
  P(t)_x : Outport
  P(t)_Omega : Outport  Port=2
  P(t)_Phi : Outport  Port=3
  P : Outport  Port=4
  wires:
  Gain1/1 -> P(t)_Phi/1
  Gain/1 -> P(t)_Omega/1
  Dot Product3/1 -> P(t)_x/1  "P"
  Dot Product2/1 -> Gain1/1  "P"
  Subtract2/1 -> Dot Product1/2, Dot Product2/2, P/1, Dot Product3/2  "P"
  Dot Product5/1 -> Abs/1
  Discrete Derivative1/1 -> Sum2/2
  Discrete Derivative/1 -> Sum2/1
  Reset/1 -> Discrete-Time Integrator4/2, Discrete-Time Integrator3/2
  0.4/1 -> Add4/2
  0.3/1 -> Add3/2
  Saturation3/1 -> Subtract2/2, Dot Product7/2
  amp2/1 -> Dot Product5/1
  Saturation/1 -> Dot Product5/2, Subtract2/1
  Dot Product1/1 -> Gain/1  "P"
  Abs1/1 -> Dot Product6/2
  eta_0/1 -> Add3/1
  Dot Product6/1 -> 0.2/1  "eta"
  Abs/1 -> Dot Product10/2
  eta_1/1 -> Dot Product10/1, Dot Product6/1
  amp1/1 -> Dot Product1/1, Dot Product3/1, Dot Product2/1, Dot Product7/1  "eta"
  Sum2/1 -> amp2/1
  Sum1/1 -> amp1/1  "F"
  T(t)/1 -> Sum1/2, Discrete Derivative1/1
  Add3/1 -> Discrete-Time Integrator4/1
  X(t)/1 -> Discrete Derivative/1, Sum1/1
  eta_2/1 -> Add4/1
  Add4/1 -> Discrete-Time Integrator3/1
  0.1/1 -> Add3/3
  Discrete-Time Integrator4/1 -> Saturation/1, 0.3/1  "eta"
  Dot Product10/1 -> 0.1/1  "eta"
  Dot Product7/1 -> Abs1/1
  0.2/1 -> Add4/3
  Discrete-Time Integrator3/1 -> Saturation3/1, 0.4/1  "eta"

== system TestStructure/InterForceControlTask/AO1/Subsystem/Subsystem3 ==
  P(t)_x : Inport
  Omega : Inport  Port=2
  P(t)_Phi : Inport  Port=3
  Add1 : Sum
  Add2 : Sum
  Divide : Product  Inputs=*/
  Dot Product1 : DotProduct  OutDataTypeStr=Inherit: Inherit via internal rule
  Dot Product3 : DotProduct  OutDataTypeStr=Inherit: Inherit via internal rule
  Dot Product4 : DotProduct  OutDataTypeStr=Inherit: Inherit via internal rule
  Gain : Gain  Gain=3
  Gain1 : Gain  Gain=0
  Gain3 : Gain
  Gain4 : Gain  Gain=-1
  MATLAB Function : MATLAB Function  TreatAsAtomicUnit=on
  Subtract1 : Sum  Inputs=+-
  Sum : Sum  Inputs=|+-
  Trigonometric Function : Trigonometry  Operator=cos
  Trigonometric Function1 : Trigonometry
  d : Constant  Value=0
  deltaphi : Constant  Value=0
  dphi : DiscreteIntegrator  ExternalReset=falling  InitialCondition=1  SampleTime=-1  ICPrevOutput=DiscIntNeverNeededParam  ICPrevScaledInput=DiscIntNeverNeededParam
  dr : DiscreteIntegrator  ExternalReset=falling  InitialCondition=1  SampleTime=-1  ICPrevOutput=DiscIntNeverNeededParam  ICPrevScaledInput=DiscIntNeverNeededParam
  x : Outport
  Phi : Outport  Port=2
  r : Outport  Port=3
  wires:
  Gain/1 -> Add2/2
  Gain4/1 -> Dot Product3/2
  P(t)_x/1 -> Dot Product1/1
  P(t)_Phi/1 -> Gain4/1
  Trigonometric Function/1 -> Dot Product4/2, Subtract1/1, Add1/1
  d/1 -> dphi/2, dr/2
  Gain3/1 -> Sum/1
  Sum/1 -> dr/1
  Gain1/1 -> Sum/2
  dr/1 -> Gain1/1, r/1, Dot Product4/1, Divide/2
  deltaphi/1 -> MATLAB Function/2(deltaphi)
  dphi/1 -> MATLAB Function/1(phi)
  Divide/1 -> Dot Product3/1
  Subtract1/1 -> Dot Product1/2
  Dot Product3/1 -> Add2/1
  Dot Product1/1 -> Gain3/1
  Omega/1 -> Gain/1
  Trigonometric Function1/1 -> Add1/2, Subtract1/2
  Dot Product4/1 -> x/1
  MATLAB Function/1(y) -> Trigonometric Function1/1, Phi/1, Trigonometric Function/1
  Add1/1 -> Divide/1
  Add2/1 -> dphi/1

== system TestStructure/InterForceControlTask/AO1/Subsystem/Subsystem5 ==
  P(t)_x : Inport
  P(t)_Phi : Inport  Port=2
  Omega : Inport  Port=3
  Add1 : Sum
  Add2 : Sum
  Divide : Product  Inputs=*/
  Dot Product1 : DotProduct  OutDataTypeStr=Inherit: Inherit via internal rule
  Dot Product3 : DotProduct  OutDataTypeStr=Inherit: Inherit via internal rule
  Dot Product4 : DotProduct  OutDataTypeStr=Inherit: Inherit via internal rule
  Gain : Gain  Gain=4
  Gain1 : Gain  Gain=0
  Gain3 : Gain
  Gain4 : Gain  Gain=-1
  MATLAB Function : MATLAB Function  TreatAsAtomicUnit=on
  Subtract1 : Sum  Inputs=+-
  Sum : Sum  Inputs=|+-
  Trigonometric Function : Trigonometry  Operator=cos
  Trigonometric Function1 : Trigonometry
  deltaphi : Constant  Value=0
  deltaphi1 : Constant  Value=0
  dphi : DiscreteIntegrator  ExternalReset=falling  InitialCondition=1  SampleTime=-1  ICPrevOutput=DiscIntNeverNeededParam  ICPrevScaledInput=DiscIntNeverNeededParam
  dr : DiscreteIntegrator  ExternalReset=falling  InitialCondition=1  SampleTime=-1  ICPrevOutput=DiscIntNeverNeededParam  ICPrevScaledInput=DiscIntNeverNeededParam
  x : Outport
  Phi : Outport  Port=2
  r : Outport  Port=3
  wires:
  Gain/1 -> Add2/2
  Gain4/1 -> Dot Product3/2
  P(t)_x/1 -> Dot Product1/1
  P(t)_Phi/1 -> Gain4/1
  Trigonometric Function/1 -> Dot Product4/2, Subtract1/1, Add1/1
  deltaphi1/1 -> dphi/2, dr/2
  Gain3/1 -> Sum/1
  Sum/1 -> dr/1
  Gain1/1 -> Sum/2
  dr/1 -> Gain1/1, r/1, Dot Product4/1, Divide/2
  deltaphi/1 -> MATLAB Function/2(deltaphi)
  dphi/1 -> MATLAB Function/1(phi)
  Divide/1 -> Dot Product3/1
  Subtract1/1 -> Dot Product1/2
  Dot Product3/1 -> Add2/1
  Dot Product1/1 -> Gain3/1
  Omega/1 -> Gain/1
  Trigonometric Function1/1 -> Add1/2, Subtract1/2
  Dot Product4/1 -> x/1
  MATLAB Function/1(y) -> Trigonometric Function1/1, Phi/1, Trigonometric Function/1
  Add1/1 -> Divide/1
  Add2/1 -> dphi/1

== system TestStructure/InterForceControlTask/AO1/Subsystem1/If Action Subsystem ==
  Action Port : ActionPort
  Constant : Constant
  Out1 : Outport
  wires:
  Constant/1 -> Out1/1

== system TestStructure/InterForceControlTask/AO1/Subsystem1/If Action Subsystem1 ==
  Action Port : ActionPort
  Constant : Constant  Value=0
  Out1 : Outport
  wires:
  Constant/1 -> Out1/1

== system TestStructure/InterForceControlTask/AO1/Subsystem1/If Action Subsystem2 ==
  WindowMin : Inport
  Action Port : ActionPort
  Function-Call Subsystem : Subsystem  TreatAsAtomicUnit=on
  Function-Call Subsystem1 : Subsystem  TreatAsAtomicUnit=on
  Function-Call Subsystem2 : Subsystem  TreatAsAtomicUnit=on
  If : If  IfExpression=(u1 > 0.4)  ElseIfExpressions=(u1< -0.4)
  Merge : Merge  Inputs=3
  Out1 : Outport
  wires:
  Function-Call Subsystem2/1(Out1) -> Merge/2
  If/2 -> Function-Call Subsystem2/Action
  If/3 -> Function-Call Subsystem1/Action
  WindowMin/1 -> If/1
  Function-Call Subsystem1/1(Out1) -> Merge/3
  Function-Call Subsystem/1(Out1) -> Merge/1
  Merge/1 -> Out1/1
  If/1 -> Function-Call Subsystem/Action

== system TestStructure/InterForceControlTask/AO1/Subsystem1/If Action Subsystem3 ==
  Action Port : ActionPort
  Constant : Constant  Value=0
  Out1 : Outport
  wires:
  Constant/1 -> Out1/1

== system TestStructure/InterForceControlTask/AO1/Subsystem1/Triggered Subsystem ==
  In1 : Inport
  Trigger : TriggerPort  VariantControl=(inherit)
  t-t_start : Outport
  wires:
  In1/1 -> t-t_start/1

== system TestStructure/InterForceControlTask/AO2/PhaseCorrection/Subsystem ==
  Peaks : Inport
  Constant3 : Constant
  Discrete-Time Integrator : DiscreteIntegrator  ExternalReset=rising  SampleTime=-1  ICPrevOutput=DiscIntNeverNeededParam  ICPrevScaledInput=DiscIntNeverNeededParam
  If : If  IfExpression=u1 == 1
  If Action Subsystem : Subsystem  TreatAsAtomicUnit=on
  If Action Subsystem1 : Subsystem  TreatAsAtomicUnit=on
  Merge : Merge
  t-t_start : Outport
  wires:
  If Action Subsystem/1(Out1) -> Merge/1
  If Action Subsystem1/1(Out1) -> Merge/2
  Constant3/1 -> Discrete-Time Integrator/1
  If/1 -> If Action Subsystem/Action
  Merge/1 -> Discrete-Time Integrator/2
  If/2 -> If Action Subsystem1/Action
  Peaks/1 -> If/1
  Discrete-Time Integrator/1 -> t-t_start/1

== system TestStructure/InterForceControlTask/AO2/PhaseCorrection/Subsystem1 ==
  Peaks : Inport
  Phi_GP(t) : Inport  Port=2
  If : If  IfExpression=u1 == 1
  If Action Subsystem : Subsystem  TreatAsAtomicUnit=on
  If Action Subsystem1 : Subsystem  TreatAsAtomicUnit=on
  Merge : Merge
  Triggered Subsystem : Subsystem  TreatAsAtomicUnit=on
  Phi_GP(t_start) : Outport
  wires:
  Phi_GP(t)/1 -> Triggered Subsystem/1(Phi_GP(t))
  If Action Subsystem/1(Out1) -> Merge/1
  If Action Subsystem1/1(Out1) -> Merge/2
  If/1 -> If Action Subsystem/Action
  Merge/1 -> Triggered Subsystem/Trigger
  If/2 -> If Action Subsystem1/Action
  Peaks/1 -> If/1
  Triggered Subsystem/1(Phi_GP(t_start)) -> Phi_GP(t_start)/1

== system TestStructure/InterForceControlTask/AO2/PhaseCorrection/Subsystem2 ==
  Phi_GP(t_start) : Inport
  If : If  IfExpression=u1 < 0.5
  If Action Subsystem : Subsystem  TreatAsAtomicUnit=on
  If Action Subsystem1 : Subsystem  TreatAsAtomicUnit=on
  Merge : Merge
  P_e(t_start) : Outport
  wires:
  If Action Subsystem1/1(Out1) -> Merge/2
  If Action Subsystem/1(Out1) -> Merge/1
  If/2 -> If Action Subsystem1/Action
  If/1 -> If Action Subsystem/Action
  Phi_GP(t_start)/1 -> If Action Subsystem/1(Phi_GP(t_start)), If Action Subsystem1/1(Phi_GP(t_start)), If/1
  Merge/1 -> P_e(t_start)/1

== system TestStructure/InterForceControlTask/AO2/PhaseCorrection/Subsystem3 ==
  Peaks : Inport
  Phi_e(t) : Inport  Port=2
  If : If  IfExpression=u1 == 1
  If Action Subsystem : Subsystem  TreatAsAtomicUnit=on
  If Action Subsystem1 : Subsystem  TreatAsAtomicUnit=on
  Merge : Merge
  Triggered Subsystem : Subsystem  TreatAsAtomicUnit=on
  Phi_e(t_start) : Outport
  wires:
  Phi_e(t)/1 -> Triggered Subsystem/1(Phi_GP(t))
  If Action Subsystem/1(Out1) -> Merge/1
  If Action Subsystem1/1(Out1) -> Merge/2
  If/1 -> If Action Subsystem/Action
  Merge/1 -> Triggered Subsystem/Trigger
  If/2 -> If Action Subsystem1/Action
  Peaks/1 -> If/1
  Triggered Subsystem/1(Phi_GP(t_start)) -> Phi_e(t_start)/1

== system TestStructure/InterForceControlTask/AO2/PhaseCorrection/Subsystem4 ==
  Reset : Inport
  0.3 : Gain  Gain=0.5
  Add3 : Sum  Inputs=+-
  Discrete-Time Integrator1 : DiscreteIntegrator  ExternalReset=falling  SampleTime=-1  ICPrevOutput=DiscIntNeverNeededParam  ICPrevScaledInput=DiscIntNeverNeededParam
  eta_0 : Constant  Value=0.5
  k_e1 : Constant
  k_e : Outport
  wires:
  Discrete-Time Integrator1/1 -> k_e/1, 0.3/1  "k_e"
  Add3/1 -> Discrete-Time Integrator1/1
  Reset/1 -> Discrete-Time Integrator1/2
  eta_0/1 -> Add3/1
  0.3/1 -> Add3/2

== system TestStructure/InterForceControlTask/AO2/PhaseCorrection/Subsystem5 ==
  Phi_e : Inport
  Phi_GP : Inport  Port=2
  Add : Sum
  Constant : Constant
  Math Function : Math  Operator=mod
  Phi_Corrected : Outport
  wires:
  Constant/1 -> Math Function/2
  Math Function/1 -> Phi_Corrected/1
  Add/1 -> Math Function/1
  Phi_GP/1 -> Add/2
  Phi_e/1 -> Add/1

== system TestStructure/InterForceControlTask/AO2/Select/If Action Subsystem ==
  Phi : Inport
  Phase0 : Inport  Port=2
  Action Port : ActionPort  InitializeStates=reset
  Counter1 : dspswit3/Counter  Direction=Up  CountEvent=Rising edge  CounterSize=8 bits  MaxCount=255  InitialCount=0  Output=Count  HitValue=32  ResetInput=off  SamplesPerFrame=1  Ts=1  CntDtype=double  HitDtype=Logical
  If : If
  If Action Subsystem : Subsystem  TreatAsAtomicUnit=on
  If Action Subsystem1 : Subsystem  TreatAsAtomicUnit=on
  Merge : Merge
  Merge1 : Merge
  Phi_Out : Outport
  Phase0Event : Outport  Port=2
  wires:
  Phase0/1 -> If Action Subsystem/2(Phase0), Counter1/1
  Phi/1 -> If Action Subsystem/1(Phi)
  Counter1/1 -> If/1
  Merge/1 -> Phi_Out/1
  If/1 -> If Action Subsystem/Action
  If Action Subsystem/1(Out1) -> Merge/1
  If/2 -> If Action Subsystem1/Action
  If Action Subsystem1/1(Out1) -> Merge/2
  Merge1/1 -> Phase0Event/1
  If Action Subsystem1/2(Out2) -> Merge1/2
  If Action Subsystem/2(Out2) -> Merge1/1

== system TestStructure/InterForceControlTask/AO2/Select/If Action Subsystem1 ==
  Action Port : ActionPort
  Constant : Constant  Value=0
  Constant1 : Constant  Value=0
  Out1 : Outport
  Out2 : Outport  Port=2
  wires:
  Constant1/1 -> Out2/1
  Constant/1 -> Out1/1
